simulink model "r2_digitiser_r001_noadc"  (R2012b)
(part 2 of 11)

      mask help:
      | Standard snap block, but with the following optional extras;
      |  1) Optionally delay the fabric trigger by a user-specified number of valids.
      |  2) Capture continuously after a trigger until a stop pulse is received. Data is captured into BRAM continuously, with old data being overwritten until a stop command is received. Then stop capturing when memory is filled. This enables you to get some data before and some data after the stop pulse. Use the 'tr_en_cnt' register to determine where you are in your vector. 'Addr' register's MSb now indicates 'busy capturing'.
      |  3) Optionally capture a value on an input port to a register at the same time as the first data sample.
      |  4) Implement counters using DSP48Es to save resources.
      mask init:
      | snapshot_init(gcb, ...
      |     'storage', storage, ...
      |     'dram_dimm', dram_dimm, ...
      |     'dram_clock', dram_clock, ...
      |     'nsamples', nsamples, ...
      |     'data_width', data_width, ...
      |     'offset', offset, ...
      |     'circap', circap, ...
      |     'value', value, ...
      |     'use_dsp48', use_dsp48);
      mask TypeOptions storage: bram | dram
      mask Callback storage: snapshot_callback();
      mask TypeOptions dram_dimm: 1 | 2 | 3 | 4
      mask TypeOptions dram_clock: 200 | 250 | 266 | 300 | 333
      mask TypeOptions data_width: 8 | 16 | 32 | 64 | 128
  spead_pack00 : Subsystem  Tag=casper:spead_pack  AncestorBlock=casper_library_communications/spead_pack  mask(pkt_pack_mask){payload_length=640, header_ids=[5632 12545 12546], spead_msw=64, spead_lsw=48, spead_version=4}
      mask prompts: payload_length "Payload Length in 64-bit words"; header_ids "SPEAD header IDs (decimal)"; spead_msw "SPEAD Flavour (MSw)"; spead_lsw "SPEAD Flavour (LSw)"; spead_version "SPEAD version"
      mask help:
      | This block generates SPEAD-compliant packets from a datastream.
      |
      | Packets are created with a fixed header followed by a number of 64-bit items.
      |
      | Requires a 64-bit data stream.
      |
      | See the documentation for further details.
      mask init:
      | spead_pack_init(gcb, header_ids)
  spead_pack01 : Subsystem  Tag=casper:spead_pack  AncestorBlock=casper_library_communications/spead_pack  mask(pkt_pack_mask){payload_length=640, header_ids=[5632 12545 12546], spead_msw=64, spead_lsw=48, spead_version=4}
      mask prompts: payload_length "Payload Length in 64-bit words"; header_ids "SPEAD header IDs (decimal)"; spead_msw "SPEAD Flavour (MSw)"; spead_lsw "SPEAD Flavour (LSw)"; spead_version "SPEAD version"
      mask help:
      | This block generates SPEAD-compliant packets from a datastream.
      |
      | Packets are created with a fixed header followed by a number of 64-bit items.
      |
      | Requires a 64-bit data stream.
      |
      | See the documentation for further details.
      mask init:
      | spead_pack_init(gcb, header_ids)
  spead_pack10 : Subsystem  Tag=casper:spead_pack  AncestorBlock=casper_library_communications/spead_pack  mask(pkt_pack_mask){payload_length=640, header_ids=[5632 12545 12546], spead_msw=64, spead_lsw=48, spead_version=4}
      mask prompts: payload_length "Payload Length in 64-bit words"; header_ids "SPEAD header IDs (decimal)"; spead_msw "SPEAD Flavour (MSw)"; spead_lsw "SPEAD Flavour (LSw)"; spead_version "SPEAD version"
      mask help:
      | This block generates SPEAD-compliant packets from a datastream.
      |
      | Packets are created with a fixed header followed by a number of 64-bit items.
      |
      | Requires a 64-bit data stream.
      |
      | See the documentation for further details.
      mask init:
      | spead_pack_init(gcb, header_ids)
  spead_pack11 : Subsystem  Tag=casper:spead_pack  AncestorBlock=casper_library_communications/spead_pack  mask(pkt_pack_mask){payload_length=640, header_ids=[5632 12545 12546], spead_msw=64, spead_lsw=48, spead_version=4}
      mask prompts: payload_length "Payload Length in 64-bit words"; header_ids "SPEAD header IDs (decimal)"; spead_msw "SPEAD Flavour (MSw)"; spead_lsw "SPEAD Flavour (LSw)"; spead_version "SPEAD version"
      mask help:
      | This block generates SPEAD-compliant packets from a datastream.
      |
      | Packets are created with a fixed header followed by a number of 64-bit items.
      |
      | Requires a 64-bit data stream.
      |
      | See the documentation for further details.
      mask init:
      | spead_pack_init(gcb, header_ids)
  spead_unpack : Subsystem  Tag=casper:spead_unpack  AncestorBlock=casper_library_communications/spead_unpack  mask(spead_unpack_mask){payload_length=640, header_ids=[5632 12545 12546], spead_msw=64, spead_lsw=48, spead_version=4, combine_errors=on}
      mask prompts: payload_length "Payload length in 64-bit words"; header_ids "SPEAD header IDs (decimal)"; spead_msw "SPEAD Flavour (MSw)"; spead_lsw "SPEAD Flavour (LSw)"; spead_version "SPEAD version"; combine_errors "Combine error flags"
      mask help: This block receives a 64-bit-word stream that contains a SPEAD stream. It checks the SPEAD headers are being correctly received. It presents the user with all headers on the first valid cycle of data along with a flag to indicate a header or packet-length error.
      mask init:
      | spead_unpack_init(gcb)
  ticks_since_mrst : Subsystem
  tvg : Subsystem
  unpack_64_to_80_1 : Subsystem
  xsg : xps_library/XSG core config  Tag=xps:xsg  hw_sys=ROACH2:sx475t  clk_src=sys_clk  ROACH_clk_src=sys_clk  ROACH2_clk_src=sys_clk  clk_rate=1712/8  sample_period=1  synthesis_tool=XST
  tag scope: local_time=global, spead_time=global
  wires:
  [mrst] -> tvg/1(reset)
  [mrst] -> ticks_since_mrst/1(reset)
  [sync] -> ticks_since_mrst/2(sync)
  ticks_since_mrst/1(time) -> slice5/1, [local_time]  "localtime"
  Logical3/1 -> [sync]  "sync"
  edge_detect2/1(out) -> [mrst]  "mrst"
  edge_detect1/1(out) -> [msync]  "msync"
  edge_detect4/1(out) -> [clr_status]  "clr_status"
  [msync] -> Logical3/2, Logical3/1
  [local_time] -> fifo_select/1(localtime)
  fifo_select/1(select) -> [fifoselect]  "fifoselect"
  tvg/1(tvg_data80_0) -> Mux/3  "tvgdata80"
  Counter Free-Running/1 -> Relational Operator1/2, Relational Operator/2
  [data80_0] -> fifo01/1(data80), fifo00/1(data80)
  [fifoselect] -> fifo00/2(fifo_we_en), Inverter/1
  [adc_data80_0] -> Mux/2
  [tvg_select0] -> Mux/1
  Mux/1 -> [data80_0]  "d80_0"
  [adc_data80_1] -> Mux1/2
  Mux1/1 -> [data80_1]  "d80_1"
  fifo00/1(fifo_data) -> pack_80_64_00/1(data80)  "data00"
  fifo00/2(fifo_dv) -> pack_80_64_00/2(valid80)  "dv00"
  fifo00/3(word_start) -> pack_80_64_00/3(word_start)  "ws00"
  fifo00/4(pkt_start) -> pack_80_64_00/4(pkt_start)  "ps00"
  spead_pack00/1(data_out) -> bus_expand1/1(bus_in), [d64_00], Delay10/1  "packd"
  spead_pack00/2(valid_out) -> Gateway Out4/1, [v64_00], Delay1/1  "packv"
  [gbe_reset] -> gbe00/1
  [gbe_enable] -> Logical2/2
  Logical2/1 -> gbe00/3
  [gbe_port00] -> gbe00/5
  Constant8/1 -> gbe00/8, gbe00/7
  gbe00/1 -> Subsystem3/1(link_up)  "ledup"
  gbe00/2 -> Terminator13/1
  gbe00/3 -> Subsystem3/3(led_tx)  "tx00"
  gbe00/4 -> gbe_stat00/5(full), Subsystem3/4(tx_full)  "full00"
  gbe00/5 -> Subsystem3/5(tx_over), gbe_stat00/6(overflow)  "over00"
  gbe00/12 -> Terminator7/1
  gbe00/11 -> Terminator6/1
  gbe00/6 -> Terminator1/1
  gbe00/8 -> Terminator3/1
  gbe00/9 -> Terminator4/1
  gbe00/10 -> Terminator5/1
  gbe00/7 -> Terminator2/1
  gbe_stat00/1(tx_cnt) -> Delay14/1(d)
  gbe_stat00/2(err_cnt) -> Delay64/1(d)
  gbetx_errcnt00/1(sim_out) -> Terminator9/1
  Delay64/1(q) -> gbetx_errcnt00/1(out_reg)
  Constant11/1 -> gbe_stat00/2(discard)
  Delay2/1 -> Subsystem3/8(eof_in), gbe_stat00/3(eof), gbe00/6
  Delay1/1 -> Subsystem3/6(valid_in), gbe_stat00/4(valid), Logical2/1
  gbetx_cnt00/1(sim_out) -> Terminator8/1
  Delay14/1(q) -> gbetx_cnt00/1(out_reg)
  [clr_status] -> gbe_stat00/1(rst)
  Delay3/1(q) -> gbetx_fullcnt00/1(out_reg)
  Delay4/1(q) -> gbetx_ofcnt00/1(out_reg)
  gbetx_ofcnt00/1(sim_out) -> Terminator11/1
  gbetx_fullcnt00/1(sim_out) -> Terminator10/1
  gbe_port/1(in_reg) -> [gbe_port10], [gbe_port01], [gbe_port00], [gbe_port11]
  gbe_ip00/1(in_reg) -> [gbe_ip00]
  gbe_ip01/1(in_reg) -> [gbe_ip01]
  gbe_ip10/1(in_reg) -> [gbe_ip10]
  gbe_ip11/1(in_reg) -> [gbe_ip11]
  Constant9/1 -> gbe_port/1(sim_1)
  Constant10/1 -> gbe_ip00/1(sim_1)
  Constant12/1 -> gbe_ip01/1(sim_1)
  Constant13/1 -> gbe_ip10/1(sim_1)
  Constant14/1 -> gbe_ip11/1(sim_1)
  Constant15/1 -> id1/1(sim_1)
  Constant17/1 -> id2/1(sim_1)
  bus_create/1(bus_out) -> [hdr_0x3101]
  Subsystem3/1(data_out) -> bus_create5/1(in1)
  Subsystem3/2(we_out) -> bus_create5/2(in2)
  Subsystem3/3(trig_out) -> bus_create5/3(in3)
  pack_80_64_00/3(data64) -> spead_pack00/3(data64)  "d64_00"
  pack_80_64_00/2(valid64) -> spead_pack00/2(data64_valid)  "v64_00"
  pack_80_64_00/1(ready64) -> spead_pack00/1(data64_ready)  "r64_00"
  fifo00/5(fifo_full) -> Terminator16/1
  fifo00/6(fifo_empty) -> Terminator23/1
  Delay10/1 -> Subsystem3/2(data_in), gbe00/2
  [gbe_ip00] -> Subsystem3/7(ip_in), gbe00/4
  gbe_stat00/3(full_count) -> Delay3/1(d)
  gbe_stat00/4(of_count) -> Delay4/1(d)
  fifo01/1(fifo_data) -> pack_80_64_01/1(data80)  "data01"
  fifo01/2(fifo_dv) -> pack_80_64_01/2(valid80)  "dv01"
  fifo01/3(word_start) -> pack_80_64_01/3(word_start)  "ws01"
  fifo01/4(pkt_start) -> pack_80_64_01/4(pkt_start)  "ps01"
  spead_pack01/1(data_out) -> bus_expand2/1(bus_in), Delay6/1
  spead_pack01/2(valid_out) -> Gateway Out2/1, Delay5/1
  spead_pack01/3(eof) -> Gateway Out6/1, Delay8/1
  [gbe_reset] -> gbe01/1
  [gbe_enable] -> Logical1/2
  Logical1/1 -> gbe01/3
  [gbe_port01] -> gbe01/5
  Constant22/1 -> gbe01/7, gbe01/8
  gbe01/1 -> Subsystem1/1(link_up)  "ledup"
  gbe01/2 -> Terminator17/1
  gbe01/3 -> Subsystem1/3(led_tx)  "tx00"
  gbe01/4 -> Subsystem1/4(tx_full), gbe_stat01/5(full)  "full00"
  gbe01/5 -> Subsystem1/5(tx_over), gbe_stat01/6(overflow)  "over00"
  gbe01/12 -> Terminator26/1
  gbe01/11 -> Terminator25/1
  gbe01/6 -> Terminator14/1
  gbe01/8 -> Terminator21/1
  gbe01/9 -> Terminator22/1
  gbe01/10 -> Terminator24/1
  gbe01/7 -> Terminator19/1
  gbe_stat01/1(tx_cnt) -> Delay7/1(d)
  gbe_stat01/2(err_cnt) -> Delay12/1(d)
  gbetx_errcnt01/1(sim_out) -> Terminator30/1
  Delay12/1(q) -> gbetx_errcnt01/1(out_reg)
  Constant20/1 -> gbe_stat01/2(discard)
  Delay8/1 -> gbe01/6, Subsystem1/8(eof_in), gbe_stat01/3(eof)
  Delay5/1 -> Logical1/1, Subsystem1/6(valid_in), gbe_stat01/4(valid)
  gbetx_cnt01/1(sim_out) -> Terminator29/1
  Delay7/1(q) -> gbetx_cnt01/1(out_reg)
  [clr_status] -> gbe_stat01/1(rst)
  Delay9/1(q) -> gbetx_fullcnt01/1(out_reg)
  Delay11/1(q) -> gbetx_ofcnt01/1(out_reg)
  gbetx_ofcnt01/1(sim_out) -> Terminator28/1
  gbetx_fullcnt01/1(sim_out) -> Terminator27/1
  spead_pack01/4(data_overflow) -> Terminator15/1
  Subsystem1/1(data_out) -> bus_create6/1(in1)
  Subsystem1/2(we_out) -> bus_create6/2(in2)
  Subsystem1/3(trig_out) -> bus_create6/3(in3)
  pack_80_64_01/3(data64) -> spead_pack01/3(data64)  "d64_00"
  pack_80_64_01/2(valid64) -> spead_pack01/2(data64_valid)  "v64_00"
  pack_80_64_01/1(ready64) -> spead_pack01/1(data64_ready)  "r64_00"
  fifo01/5(fifo_full) -> Terminator18/1
  fifo01/6(fifo_empty) -> Terminator20/1
  Delay6/1 -> Subsystem1/2(data_in), gbe01/2
  [gbe_ip01] -> Subsystem1/7(ip_in), gbe01/4
  gbe_stat01/3(full_count) -> Delay9/1(d)
  gbe_stat01/4(of_count) -> Delay11/1(d)
  Inverter/1 -> fifo01/2(fifo_we_en)
  [data80_1] -> fifo11/1(data80), fifo10/1(data80)
  [fifoselect] -> fifo10/2(fifo_we_en), Inverter1/1
  fifo10/1(fifo_data) -> pack_80_64_10/1(data80)  "data00"
  fifo10/2(fifo_dv) -> pack_80_64_10/2(valid80)  "dv00"
  fifo10/3(word_start) -> pack_80_64_10/3(word_start)  "ws00"
  fifo10/4(pkt_start) -> pack_80_64_10/4(pkt_start)  "ps00"
  spead_pack10/1(data_out) -> bus_expand3/1(bus_in), Delay15/1
  spead_pack10/2(valid_out) -> Gateway Out8/1, Delay13/1
  spead_pack10/3(eof) -> Gateway Out9/1, Delay19/1
  [gbe_reset] -> gbe10/1
  [gbe_enable] -> Logical5/2
  Logical5/1 -> gbe10/3
  [gbe_port10] -> gbe10/5
  Constant29/1 -> gbe10/7, gbe10/8
  gbe10/1 -> Subsystem4/1(link_up)  "ledup"
  gbe10/2 -> Terminator35/1
  gbe10/3 -> Subsystem4/3(led_tx)  "tx00"
  gbe10/4 -> Subsystem4/4(tx_full), gbe_stat10/5(full)  "full00"
  gbe10/5 -> Subsystem4/5(tx_over), gbe_stat10/6(overflow)  "over00"
  gbe10/12 -> Terminator58/1
  gbe10/11 -> Terminator57/1
  gbe10/6 -> Terminator31/1
  gbe10/8 -> Terminator53/1
  gbe10/9 -> Terminator55/1
  gbe10/10 -> Terminator56/1
  gbe10/7 -> Terminator42/1
  gbe_stat10/1(tx_cnt) -> Delay18/1(d)
  gbe_stat10/2(err_cnt) -> Delay24/1(d)
  gbetx_errcnt10/1(sim_out) -> Terminator60/1
  Delay24/1(q) -> gbetx_errcnt10/1(out_reg)
  Constant24/1 -> gbe_stat10/2(discard)
  Delay19/1 -> gbe10/6, Subsystem4/8(eof_in), gbe_stat10/3(eof)
  Delay13/1 -> Logical5/1, Subsystem4/6(valid_in), gbe_stat10/4(valid)
  gbetx_cnt10/1(sim_out) -> Terminator59/1
  Delay18/1(q) -> gbetx_cnt10/1(out_reg)
  [clr_status] -> gbe_stat10/1(rst)
  Delay20/1(q) -> gbetx_fullcnt10/1(out_reg)
  Delay21/1(q) -> gbetx_ofcnt10/1(out_reg)
  gbetx_ofcnt10/1(sim_out) -> Terminator33/1
  gbetx_fullcnt10/1(sim_out) -> Terminator32/1
  spead_pack10/4(data_overflow) -> Terminator34/1
  Subsystem4/1(data_out) -> bus_create7/1(in1)
  Subsystem4/2(we_out) -> bus_create7/2(in2)
  Subsystem4/3(trig_out) -> bus_create7/3(in3)
  pack_80_64_10/3(data64) -> spead_pack10/3(data64)  "d64_00"
  pack_80_64_10/2(valid64) -> spead_pack10/2(data64_valid)  "v64_00"
  pack_80_64_10/1(ready64) -> spead_pack10/1(data64_ready)  "r64_00"
  fifo10/5(fifo_full) -> Terminator38/1
  fifo10/6(fifo_empty) -> Terminator46/1
  Delay15/1 -> Subsystem4/2(data_in), gbe10/2
  [gbe_ip10] -> Subsystem4/7(ip_in), gbe10/4
  gbe_stat10/3(full_count) -> Delay20/1(d)
  gbe_stat10/4(of_count) -> Delay21/1(d)
  fifo11/1(fifo_data) -> pack_80_64_11/1(data80)  "data00"
  fifo11/2(fifo_dv) -> pack_80_64_11/2(valid80)  "dv00"
  fifo11/3(word_start) -> pack_80_64_11/3(word_start)  "ws00"
  fifo11/4(pkt_start) -> pack_80_64_11/4(pkt_start)  "ps00"
  spead_pack11/1(data_out) -> bus_expand4/1(bus_in), Delay23/1
  spead_pack11/2(valid_out) -> Gateway Out11/1, Delay22/1
  spead_pack11/3(eof) -> Gateway Out12/1, Delay26/1
  [gbe_reset] -> gbe11/1
  [gbe_enable] -> Logical4/2
  Logical4/1 -> gbe11/3
  [gbe_port11] -> gbe11/5
  Constant28/1 -> gbe11/8, gbe11/7
  gbe11/1 -> Subsystem2/1(link_up)  "ledup"
  gbe11/2 -> Terminator39/1
  gbe11/3 -> Subsystem2/3(led_tx)  "tx00"
  gbe11/4 -> Subsystem2/4(tx_full), gbe_stat11/5(full)  "full00"
  gbe11/5 -> Subsystem2/5(tx_over), gbe_stat11/6(overflow)  "over00"
  gbe11/12 -> Terminator49/1
  gbe11/11 -> Terminator48/1
  gbe11/6 -> Terminator36/1
  gbe11/8 -> Terminator44/1
  gbe11/9 -> Terminator45/1
  gbe11/10 -> Terminator47/1
  gbe11/7 -> Terminator41/1
  gbe_stat11/1(tx_cnt) -> Delay25/1(d)
  gbe_stat11/2(err_cnt) -> Delay17/1(d)
  gbetx_errcnt11/1(sim_out) -> Terminator54/1
  Delay17/1(q) -> gbetx_errcnt11/1(out_reg)
  Constant26/1 -> gbe_stat11/2(discard)
  Delay26/1 -> Subsystem2/8(eof_in), gbe_stat11/3(eof), gbe11/6
  Delay22/1 -> Subsystem2/6(valid_in), gbe_stat11/4(valid), Logical4/1
  gbetx_cnt11/1(sim_out) -> Terminator52/1
  Delay25/1(q) -> gbetx_cnt11/1(out_reg)
  [clr_status] -> gbe_stat11/1(rst)
  Delay27/1(q) -> gbetx_fullcnt11/1(out_reg)
  Delay16/1(q) -> gbetx_ofcnt11/1(out_reg)
  gbetx_ofcnt11/1(sim_out) -> Terminator51/1
  gbetx_fullcnt11/1(sim_out) -> Terminator50/1
  spead_pack11/4(data_overflow) -> Terminator37/1
  Subsystem2/1(data_out) -> bus_create8/1(in1)
  Subsystem2/2(we_out) -> bus_create8/2(in2)
  Subsystem2/3(trig_out) -> bus_create8/3(in3)
  pack_80_64_11/3(data64) -> spead_pack11/3(data64)  "d64_00"
  pack_80_64_11/2(valid64) -> spead_pack11/2(data64_valid)  "v64_00"
  pack_80_64_11/1(ready64) -> spead_pack11/1(data64_ready)  "r64_00"
  fifo11/5(fifo_full) -> Terminator40/1
  fifo11/6(fifo_empty) -> Terminator43/1
  Delay23/1 -> Subsystem2/2(data_in), gbe11/2
  [gbe_ip11] -> Subsystem2/7(ip_in), gbe11/4
  gbe_stat11/3(full_count) -> Delay27/1(d)
  gbe_stat11/4(of_count) -> Delay16/1(d)
  Inverter1/1 -> fifo11/2(fifo_we_en)
  bus_create5/1(bus_out) -> [snap_tx00]
  bus_create6/1(bus_out) -> [snap_tx01]
  bus_create7/1(bus_out) -> [snap_tx10]
  bus_create8/1(bus_out) -> [snap_tx11]
  bus_expand/1(msb_out3) -> snap_gbe_tx/1(din)
  bus_expand/2(out2) -> snap_gbe_tx/2(we)
  bus_expand/3(lsb_out1) -> snap_gbe_tx/3(trig)
  Mux2/1 -> bus_expand/1(bus_in)
  [snap_tx_sel] -> Mux2/1
  [snap_tx00] -> Mux2/2
  [snap_tx10] -> Mux2/4
  [snap_tx01] -> Mux2/3
  [snap_tx11] -> Mux2/5
  [grng_data80] -> Mux1/4
  [grng_data80] -> Mux/4
  [tvg_select1] -> Mux1/1
  slice5/1 -> [spead_time]  "spead_time"
  tvg/2(tvg_data80_1) -> Mux1/3
  Constant34/1 -> [grng_data80], [adc_data80_0]
  Constant35/1 -> [adc_data80_1]
  Constant36/1 -> [adc_or0]
  Constant37/1 -> [adc_or1]
  Constant38/1 -> [adc_sync0]
  Constant39/1 -> [adc_sync1]
  control/1(in_tvg_select0) -> [tvg_select0]
  control/3(in_gmg_corr) -> [grng_corr]  "gbe_enable"
  control/2(in_tvg_select1) -> [tvg_select1]
  control/4(in_gmg_reset) -> [grng_reset]  "gbe_reset"
  control/5(in_snap_tx_sel) -> [snap_tx_sel]
  control/6(in_clr_status) -> edge_detect4/1(in)
  control/7(in_gbe_reset) -> [gbe_reset]
  control/8(in_gbe_enable) -> [gbe_enable]
  control/9(in_msync) -> edge_detect1/1(in)
  control/10(in_mrst) -> edge_detect2/1(in)
  Constant16/1 -> id1/2(sim_2)
  id1/1(in_digitiser_id) -> bus_create/1(in1)
  id1/2(in_digitiser_type) -> bus_create/2(in2)
  id2/1(in_receptor_id) -> bus_create/3(in3)
  id2/2(in_pol0_id) -> [pol0_id]
  id2/3(in_pol1_id) -> [pol1_id]
  Constant6/1 -> id2/2(sim_2)
  Constant19/1 -> id2/3(sim_3)
  [hdr_0x3101] -> bus_create9/1(in1)
  [pol0_id] -> bus_create9/2(in2)
  [hdr_0x3101] -> bus_create1/1(in1)
  [pol0_id] -> bus_create1/2(in2)
  [hdr_0x3101] -> bus_create2/1(in1)
  [pol1_id] -> bus_create2/2(in2)
  [hdr_0x3101] -> bus_create3/1(in1)
  [pol1_id] -> bus_create3/2(in2)
  Relational Operator1/1 -> control/9(sim_9)
  Relational Operator/1 -> control/10(sim_10)
  Constant1/1 -> Relational Operator/1
  Constant/1 -> Relational Operator1/1
  Constant33/1 -> control/8(sim_8)
  Constant31/1 -> control/7(sim_7)
  Constant30/1 -> control/6(sim_6)
  Constant7/1 -> control/5(sim_5)
  Constant5/1 -> control/4(sim_4)
  Constant4/1 -> control/3(sim_3)
  Constant3/1 -> control/2(sim_2)
  Constant2/1 -> control/1(sim_1)
  [spead_time] -> spead_pack00/4(hdr1_0x1600)
  bus_create9/1(bus_out) -> spead_pack00/5(hdr2_0x3101)
  [status00] -> spead_pack00/6(hdr3_0x3102)
  [spead_time] -> spead_pack01/4(hdr1_0x1600)
  bus_create1/1(bus_out) -> spead_pack01/5(hdr2_0x3101)
  [status01] -> spead_pack01/6(hdr3_0x3102)
  [spead_time] -> spead_pack10/4(hdr1_0x1600)
  bus_create2/1(bus_out) -> spead_pack10/5(hdr2_0x3101)
  [status10] -> spead_pack10/6(hdr3_0x3102)
  [spead_time] -> spead_pack11/4(hdr1_0x1600)
  bus_create3/1(bus_out) -> spead_pack11/5(hdr2_0x3101)
  [status11] -> spead_pack11/6(hdr3_0x3102)
  Gateway Out4/1 -> To Workspace4/1
  Gateway Out5/1 -> To Workspace5/1
  Gateway Out2/1 -> To Workspace2/1
  Gateway Out6/1 -> To Workspace6/1
  Gateway Out8/1 -> To Workspace8/1
  Gateway Out9/1 -> To Workspace9/1
  Gateway Out11/1 -> To Workspace11/1
  Gateway Out12/1 -> To Workspace12/1
  Constant23/1 -> [status00]
  Constant18/1 -> [status01]
  Constant21/1 -> [status10]
  Constant25/1 -> [status11]
  spead_pack00/3(eof) -> [e64_00], Gateway Out5/1, Delay2/1
  spead_pack00/4(data_overflow) -> Terminator12/1
  spead_unpack/2(data64) -> unpack_64_to_80_1/2(data64)  "d64"
  spead_unpack/3(valid64) -> unpack_64_to_80_1/3(valid64)  "v64"
  spead_unpack/1(pkt_start) -> unpack_64_to_80_1/1(pkt_start)  "s64"
  unpack_64_to_80_1/1(start80) -> Terminator70/1  "s80"
  unpack_64_to_80_1/2(data80) -> Terminator73/1  "d80"
  unpack_64_to_80_1/3(valid80) -> Terminator75/1  "v80"
  unpack_64_to_80_1/4(eof80) -> Terminator76/1  "e80"
  spead_unpack/4(eof64) -> unpack_64_to_80_1/4(eof64)  "e64"
  spead_unpack/5(error) -> Terminator69/1  "err64"
  spead_unpack/6(hdr1_0x1600) -> Terminator71/1  "hdr1"
  spead_unpack/7(hdr2_0x3101) -> Terminator72/1  "hdr2"
  spead_unpack/8(hdr3_0x3102) -> Terminator74/1  "hdr3"
  [e64_00] -> spead_unpack/3(pkt_eof)
  [v64_00] -> spead_unpack/2(pkt_valid)
  [d64_00] -> spead_unpack/1(pkt_data)
  local_time_lsw/1(sim_out) -> Terminator62/1
  local_time_msw/1(sim_out) -> Terminator61/1
  [local_time] -> slice1/1, slice2/1
  slice2/1 -> local_time_msw/1(out_reg)
  slice1/1 -> local_time_lsw/1(out_reg)
